simulink model "Ej6"  (R2025a)
settings: Solver=VariableStepAuto  StartTime=0.0  StopTime=10.0  RelTol=1e-3
libraries: commrandsrc3 x1
settings Model: Creator=Henry  LastModifiedBy=Henry

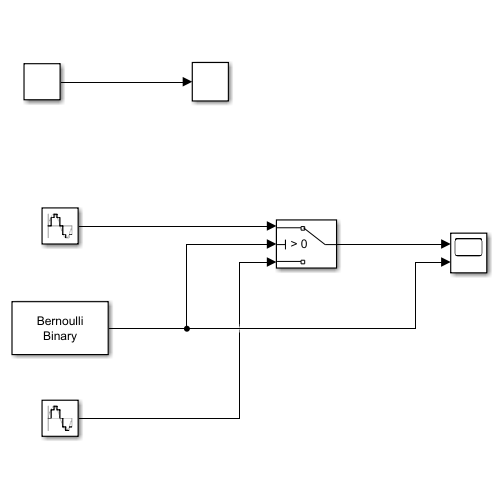
[thumbnail: Simulink's stored preview of the top-level diagram]
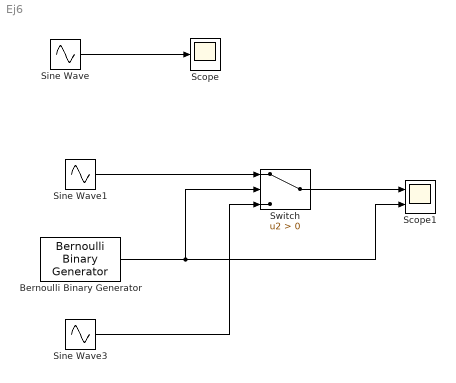
== system Ej6 ==
  Bernoulli Binary Generator : commrandsrc3/Bernoulli Binary Generator  ProbabilityOfZero=0.5  SeedSource=Auto  Seed=0  SampleTime=1  SamplesPerFrame=1  OutputDataType=double  SimulateUsing=Interpreted execution
  Scope : Scope
      settings: ActiveDisplayYMinimum=-1.2456318853205086  ActiveDisplayYMaximum=1.2490408795261734
  Scope1 : Scope  NumInputPorts=2
      settings: ActiveDisplayYMinimum=-1  ActiveDisplayYMaximum=1
  Sine Wave : Sin  SampleTime=0
  Sine Wave1 : Sin  Frequency=110*2*pi  SampleTime=0.0001
  Sine Wave3 : Sin  Frequency=2*pi*10  SampleTime=0.0001
  Switch : Switch  Criteria=u2 > Threshold  SaturateOnIntegerOverflow=off  InputSameDT=off
  wires:
  Sine Wave/1 -> Scope/1
  Sine Wave1/1 -> Switch/1
  Bernoulli Binary Generator/1 -> Scope1/2, Switch/2
  Sine Wave3/1 -> Switch/3
  Switch/1 -> Scope1/1
